simulink model "fractional_4"  (Simulink 7.4)
settings: Solver=ode45  StartTime=0.0  StopTime=1.6e-5  FixedStep=.01/(fr*N/M)  MaxStep=1/(25*fr*N)  RelTol=1e-5  AbsTol=1e-4
PreLoadFcn:
  | fr=10e6,fi=90e6,sen=10e6,N=10,M=.1
  | D=8;
StartFcn:
  | tic;
StopFcn:
  | trun=toc
undefined symbols (not defined in the file or in its folder): M, N, One, sen, sided
libraries: dspsigops x5, simulink_extras x5, dspsigattribs x4, simulink x3, dspstat3 x2, commblksprivate x2, dspsnks4 x1, dsparch4 x1
settings Model: Creator=rab  LastModifiedBy=Dick  BufferReuse=off
settings Model: ModifiedHistory=|
  | phase error compensation and swallow counter
  | incorporated by Benson,  Fall 2001.
settings DataIOCC: LimitDataPoints=off  SaveOutput=off  SaveTime=off  SignalLoggingName=sigsOut
settings OptimizationCC: BlockReduction=off  BooleanDataType=off  InlineInvariantSignals=on  OptimizeBlockIOStorage=off  BufferReuse=off  ExpressionFolding=off  LocalBlockOutputs=off  InitFltsAndDblsToZero=on
settings DebuggingCC: SaveWithParameterizedLinksMsg=none  SignalResolutionControl=TryResolveAllWithWarning  SolverPrmCheckMsg=none  MultiTaskDSMMsg=warning  MultiTaskCondExecSysMsg=none  StrictBusMsg=None
settings HardwareCC: TargetUnknown=on
settings RTWCC: IncludeERTFirstTime=on
settings GRTTargetCC: TargetFcnLib=ansi_tfl_tmw.mat

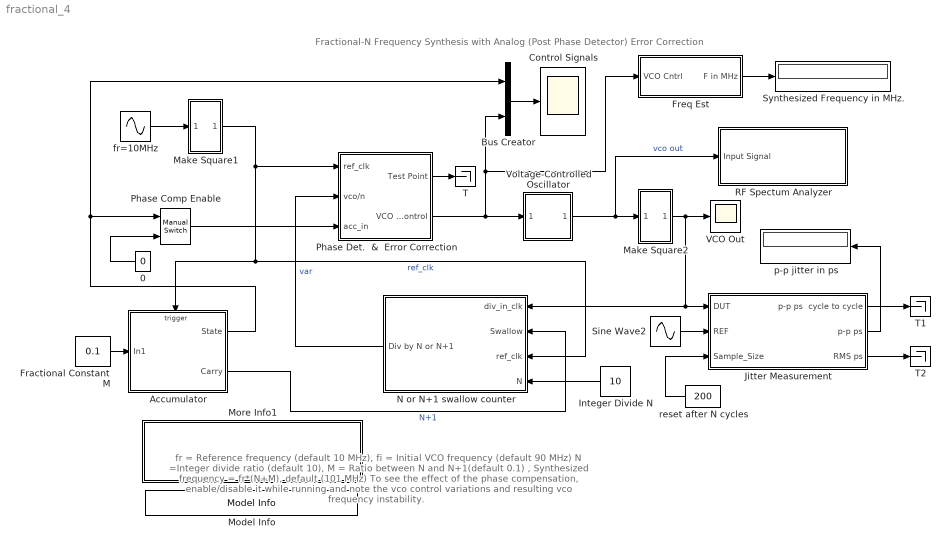
== system fractional_4 ==
  note: Fractional-N Frequency Synthesis with Analog (Post Phase Detector) Error Correction
  note: fr = Reference frequency (default 10 MHz),  fi = Initial VCO frequency (default 90 MHz)
      | N =Integer divide ratio (default 10),  M = Ratio between N and N+1(default 0.1) ,
      | Synthesized frequency = fr*(N+M), default (101 MHz)
      | To see the effect of the phase compensation, enable/disable it while running and note the vco control
      | variations and resulting vco frequency instability.
  0 : Constant  Value=0  OutDataType=sfix(16)  OutScaling=2^0
  Accumulator : Subsystem  TreatAsAtomicUnit=on
  Bus Creator : BusCreator  Inputs=2
  Control Signals : Scope
      settings: TimeRange=1.6e-005  YMin=-0.2  YMax=1.4  MaxDataPoints=60000
  Fractional Constant  M : Constant  Value=0.1  OutDataType=sfix(16)  OutScaling=2^0
  Freq Est : Subsystem
  Integer Divide N : Constant  Value=10  OutDataType=sfix(16)  OutScaling=2^0
  "Jitter Measurement " : Subsystem
  Make Square1 : Subsystem
      mask Type: Make Square
      mask Description:
      | For input +ve values output is 1
      | For input -ve values output is 0
      mask Display: plot(0,0,100,100,[90,70,70,50,50,30,30,10,10],[20,20,40,40,20,20,40,40,20],[90,87,84,80,76,73,70,67,63,60,57,53,50,47,44,40,36,33,30,27,23,20,17,13,10],[70,65,63,62,63,65,70,75,77,78,77,75,70,65,63,62,63,65,70,75,77,78,77,75,70])
  Make Square2 : Subsystem
      mask Type: Make Square
      mask Description:
      | For input +ve values output is 1
      | For input -ve values output is 0
      mask Display: plot(0,0,100,100,[90,70,70,50,50,30,30,10,10],[20,20,40,40,20,20,40,40,20],[90,87,84,80,76,73,70,67,63,60,57,53,50,47,44,40,36,33,30,27,23,20,17,13,10],[70,65,63,62,63,65,70,75,77,78,77,75,70,65,63,62,63,65,70,75,77,78,77,75,70])
  Model Info : simulink/Model-Wide Utilities/Model Info  SystemSampleTime=-1  InitialBlockCM=none  BlockCM=none  Frame=on  DisplayStringWithTags=Copywrite 2005-2010 The MathWorks, Inc.  HorizontalTextAlignment=Center  LeftAlignmentValue=0.5  SourceBlockDiagram=fractional_4  TagMaxNumber=20
  More Info1 : Subsystem
      mask Display: disp('Fractional N PLL with\n Analog Phase Correction\n Info ')
  N or N+1 swallow counter : Subsystem
  Phase Comp Enable : simulink/Signal Routing/Manual Switch  SystemSampleTime=-1  sw=1  action=0  varsize=off
  Phase Det.  &  Error Correction : Subsystem  mask{K=1.0}
      mask prompts: K "K="
      mask Display: disp('Phase Det')
  RF Spectum Analyzer : Subsystem  Description=Spectrum Analyzer  mask{BW=20e6, Fc=fr*(M+N)}
      mask prompts: BW "Bandwidth"; Fc "Center Freq"
      mask Display: fprintf('Spectrum Analyzer \n Fc=%7.2f MHz \n BW=%7.2f MHz',Fc/1e6,BW/1e6)
  Sine Wave2 : Sin  Amplitude=1  Bias=0  Frequency=2*pi*fr*(N+M)  Phase=0  Samples=10  SampleTime=0  Offset=0
  Synthesized Frequency in MHz. : Display
      settings: Decimation=401
  T : Terminator
  T1 : Terminator
  T2 : Terminator
  VCO Out : Scope
      settings: TimeRange=9.900990099009902e-009  YMin=-0.1  YMax=1.1  MaxDataPoints=500
  Voltage-Controlled Oscillator : Subsystem  mask(Voltage-Controlled Oscillator){Ac=1, Fc=fi, Kc=sen, Ph=0}
      mask prompts: Ac "Output amplitude:"; Fc "Oscillation frequency (Hz):"; Kc "Input sensitivity:"; Ph "Initial phase (rad):"
      mask help: Generate a continuous-time output signal whose frequency changes in response to the amplitude variations of the input signal. The input signal must be a sample-based scalar.
      mask init:
      | if ((length(Ac)~=1) | (length(Fc)~=1) | (length(Ph)~=1) | (length(Kc)~=1) )error('Mask parameters must be scalar values.');end;
      | pi2=2*pi;
      mask Help: helpview(commbhelp)
      mask Display: disp('VCO')
  fr=10MHz : Sin  Amplitude=1  Bias=0  Frequency=2*pi*fr  Phase=pi  Samples=10  SampleTime=0  Offset=0
  p-p jitter in ps : Display
  reset after N cycles : Constant  Value=200  VectorParams1D=off  OutDataType=sfix(16)  OutScaling=2^0
  wires:
  N or N+1 swallow counter/1(Div by N or N+1) -> Phase Det.  &  Error Correction/2(vco/n)  "var"
  Fractional Constant  M/1 -> Accumulator/1(In1)
  Make Square2/1(Out1) -> VCO Out/1, N or N+1 swallow counter/1(div_in_clk), "Jitter Measurement "/1(DUT)
  Accumulator/2(Carry) -> N or N+1 swallow counter/2(Swallow)  "N+1"
  Integer Divide N/1 -> N or N+1 swallow counter/4(N)
  0/1 -> Phase Comp Enable/2
  Freq Est/1(F in MHz) -> Synthesized Frequency in MHz./1
  Sine Wave2/1 -> "Jitter Measurement "/2(REF)
  "Jitter Measurement "/2(p-p ps) -> p-p jitter in ps/1
  reset after N cycles/1 -> "Jitter Measurement "/3(Sample_Size)
  Bus Creator/1 -> Control Signals/1
  Accumulator/1(State) -> Phase Comp Enable/1, Bus Creator/1
  Make Square1/1(Out1) -> Accumulator/Trigger, N or N+1 swallow counter/3(ref_clk), Phase Det.  &  Error Correction/1(ref_clk)  "ref_clk"
  Phase Comp Enable/1 -> Phase Det.  &  Error Correction/3("acc_in ")
  Voltage-Controlled Oscillator/1(out_1) -> Make Square2/1(In1), RF Spectum Analyzer/1(Input Signal)  "vco out"
  Phase Det.  &  Error Correction/2(VCO Control) -> Freq Est/1(VCO Cntrl), Bus Creator/2, Voltage-Controlled Oscillator/1(in_1)
  fr=10MHz/1 -> Make Square1/1(In1)
  Phase Det.  &  Error Correction/1(Test Point) -> T/1
  "Jitter Measurement "/1(p-p ps  cycle to cycle) -> T1/1
  "Jitter Measurement "/3(RMS ps) -> T2/1

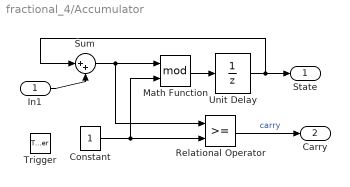
== system fractional_4/Accumulator ==
  In1 : Inport  OutDataType=sfix(16)  OutScaling=2^0
  Trigger : TriggerPort
  Constant : Constant  OutDataType=sfix(16)  OutScaling=2^0
  Math Function : Math  Operator=mod  OutDataType=sfix(16)  OutScaling=2^0  SaturateOnIntegerOverflow=on
  Relational Operator : RelationalOperator  InputSameDT=on
  Sum : Sum  Inputs=|++  OutDataType=sfix(16)  OutScaling=2^0  SaturateOnIntegerOverflow=on  InputSameDT=on  OutDataTypeStr=Inherit: Same as first input
  Unit Delay : UnitDelay  SampleTime=-1
  State : Outport  OutDataType=sfix(16)  OutScaling=2^0  InitialOutput=0
  Carry : Outport  Port=2  OutDataType=sfix(16)  OutScaling=2^0
  wires:
  In1/1 -> Sum/2
  Sum/1 -> Relational Operator/1, Math Function/1
  Math Function/1 -> Unit Delay/1
  Constant/1 -> Math Function/2, Relational Operator/2
  Relational Operator/1 -> Carry/1  "carry"
  Unit Delay/1 -> Sum/1, State/1

== system fractional_4/Freq Est ==
  VCO Cntrl : Inport  OutDataType=sfix(16)  OutScaling=2^0
  F : Constant  Value=fi  OutDataType=sfix(16)  OutScaling=2^0
  Gain1 : Gain  Gain=1e-6  ParameterDataType=sfix(16)  ParameterScaling=2^0  OutDataType=sfix(16)  OutScaling=2^0  SaturateOnIntegerOverflow=on  OutDataTypeStr=Inherit: Same as input  ParamDataTypeStr=Inherit: Same as input
  Gain3 : Gain  Gain=sen  ParameterDataType=sfix(16)  ParameterScaling=2^0  OutDataType=sfix(16)  OutScaling=2^0  SaturateOnIntegerOverflow=on  OutDataTypeStr=Inherit: Same as input  ParamDataTypeStr=Inherit: Same as input
  Sum1 : Sum  Inputs=|++  OutDataType=sfix(16)  OutScaling=2^0  SaturateOnIntegerOverflow=on  InputSameDT=on  OutDataTypeStr=Inherit: Same as first input
  F in MHz : Outport  OutDataType=sfix(16)  OutScaling=2^0
  wires:
  Sum1/1 -> Gain1/1
  F/1 -> Sum1/2
  Gain3/1 -> Sum1/1
  VCO Cntrl/1 -> Gain3/1
  Gain1/1 -> F in MHz/1

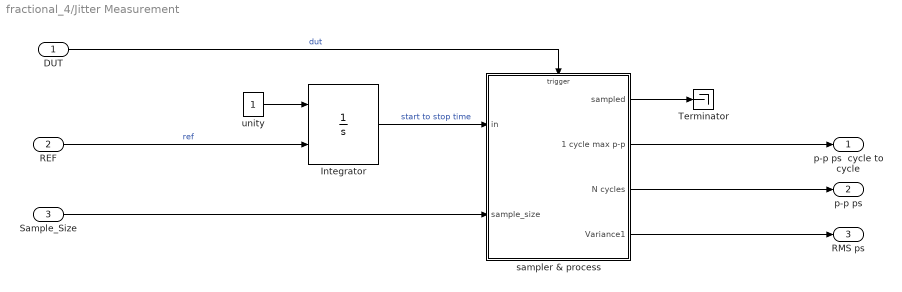
== system fractional_4/Jitter Measurement  ==
  DUT : Inport  OutDataType=sfix(16)  OutScaling=2^0
  REF : Inport  Port=2  OutDataType=sfix(16)  OutScaling=2^0
  Sample_Size : Inport  Port=3  OutDataType=sfix(16)  OutScaling=2^0
  Integrator : Integrator  ExternalReset=rising
  Terminator : Terminator
  sampler & process : Subsystem  TreatAsAtomicUnit=on
  unity : Constant  OutDataTypeMode=double  OutDataType=sfix(16)  OutScaling=2^0  OutDataTypeStr=double
  p-p ps  cycle to cycle : Outport  OutDataType=sfix(16)  OutScaling=2^0
  p-p ps : Outport  Port=2  OutDataType=sfix(16)  OutScaling=2^0
  RMS ps : Outport  Port=3  OutDataType=sfix(16)  OutScaling=2^0
  wires:
  DUT/1 -> sampler & process/Trigger  "dut"
  REF/1 -> Integrator/2  "ref"
  Integrator/1 -> sampler & process/1(in)  "start to stop time"
  Sample_Size/1 -> sampler & process/2(sample_size)
  sampler & process/3(N cycles) -> p-p ps/1
  sampler & process/4(Variance1) -> RMS ps/1
  unity/1 -> Integrator/1
  sampler & process/2(1 cycle max p-p) -> p-p ps  cycle to cycle/1
  sampler & process/1(sampled) -> Terminator/1

== system fractional_4/Make Square1 ==
  In1 : Inport  OutDataType=sfix(16)  OutScaling=2^0
  Constant : Constant  Value=0  OutDataType=sfix(16)  OutScaling=2^0
  Relational Operator : RelationalOperator  Operator=>  InputSameDT=on
  Out1 : Outport  OutDataType=sfix(16)  OutScaling=2^0
  wires:
  In1/1 -> Relational Operator/1
  Constant/1 -> Relational Operator/2
  Relational Operator/1 -> Out1/1

== system fractional_4/Make Square2 ==
  In1 : Inport  OutDataType=sfix(16)  OutScaling=2^0
  Constant : Constant  Value=0  OutDataType=sfix(16)  OutScaling=2^0
  Relational Operator : RelationalOperator  Operator=>  InputSameDT=on
  Out1 : Outport  OutDataType=sfix(16)  OutScaling=2^0
  wires:
  Relational Operator/1 -> Out1/1
  Constant/1 -> Relational Operator/2
  In1/1 -> Relational Operator/1

== system fractional_4/More Info1 ==
  note: Fractional-N PLL with Analog Phase Error Correction
  note: Fractional N PLL synthesizers attain improved frequency resolution at the expense
      | of increased circuit complexity and increased phase noise (timing jitter) over thier
      | non fractional counterparts. The average output frequency  of the PLL is (N+M)*fr where fr is
      | the frequency reference. The M term is the "fractional" part and lies between 0.0 and 1.
      |
      | This model implements a fractional N scheme with analog phase error correction
      | in the phase detector portion of the design. This *eliminates*  the sidebands introduced
      | by switching the loop divider between N and N+1.  Implementing the phase error correction
      | circuitry as part of the phase detector and loop compensation filter yeilds a design that
      | is easier to implement than the previous model that required a phase shifted clock.
      |
      |
      | 1)Phase-frequency detector and error compensator uses "dual D" flip flop phase
      | detector, integrator, sample / hold, and simple lead/lag loop filter.
      |
      | 2) Divide by N or N+1 is implemented using a "swallow" counter
      | scheme, like it would likely be done in hardware.
      |
      | 3) A modulo 1 accumulator controls the switching between N and N+1 with
      | the carry output.  The accumulator output (state) is used to drive the phase
      | compensation circuitry.
      |
      | 4) Run the simulation with the compensation off: switch in lower position.
      | Miminize the model to look at the graphs. Note the significant phase
      | jitter and sidebands due to the periodic variations of the VCO control
      | voltage.
      |
      | 5) Change the switch to the upper (compensation on) position. Note
      | the complete elimination  of  timing jitter, and, frequency spurs. Also note that
      | it is far easier to see the modulation in the frequency domain
      | sidebands  than the phase jitter of the clock.  The single remaining spur
      | (-100 dBc).
      |
      | 6) The Simulink model and simulation are virtually perfect. Real world component
      | limitations can now be introduced to study their effects on the system performance.

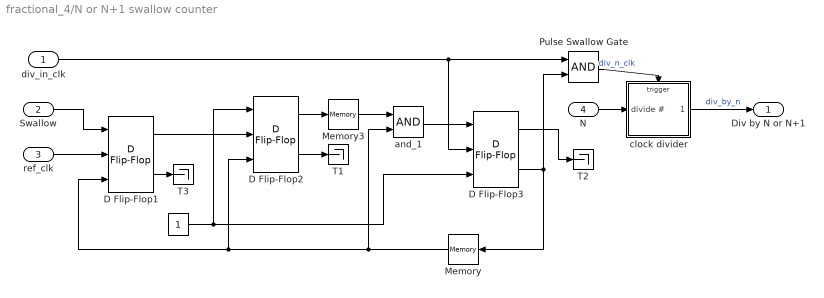
== system fractional_4/N or N+1 swallow counter ==
  div_in_clk : Inport  OutDataType=sfix(16)  OutScaling=2^0
  Swallow : Inport  Port=2  OutDataType=sfix(16)  OutScaling=2^0
  ref_clk : Inport  Port=3  OutDataType=sfix(16)  OutScaling=2^0
  N : Inport  Port=4  OutDataType=sfix(16)  OutScaling=2^0
  " " : Constant  OutDataType=sfix(16)  OutScaling=2^0
  D Flip-Flop1 : simulink_extras/Flip Flops/D Flip-Flop  SystemSampleTime=-1
  D Flip-Flop2 : simulink_extras/Flip Flops/D Flip-Flop  SystemSampleTime=-1
  D Flip-Flop3 : simulink_extras/Flip Flops/D Flip-Flop  SystemSampleTime=-1
  Memory : Memory
  Memory3 : Memory
  Pulse Swallow Gate : Logic
  T1 : Terminator
  T2 : Terminator
  T3 : Terminator
  and_1 : Logic
  clock divider : Subsystem  TreatAsAtomicUnit=on
  Div by N or N+1 : Outport  OutDataType=sfix(16)  OutScaling=2^0
  wires:
  N/1 -> clock divider/1("divide # ")
  D Flip-Flop1/2 -> T3/1
  D Flip-Flop2/2 -> T1/1
  D Flip-Flop3/1 -> T2/1
  Memory3/1 -> and_1/1
  D Flip-Flop1/1 -> D Flip-Flop2/2
  ref_clk/1 -> D Flip-Flop1/2
  Swallow/1 -> D Flip-Flop1/1
  and_1/1 -> D Flip-Flop3/1
  " "/1 -> D Flip-Flop3/3, D Flip-Flop2/1
  Memory/1 -> and_1/2, D Flip-Flop1/3, D Flip-Flop2/3
  D Flip-Flop3/2 -> Memory/1, Pulse Swallow Gate/2
  D Flip-Flop2/1 -> Memory3/1
  div_in_clk/1 -> D Flip-Flop3/2, Pulse Swallow Gate/1
  clock divider/1(" ") -> Div by N or N+1/1  "div_by_n"
  Pulse Swallow Gate/1 -> clock divider/Trigger  "div_n_clk"

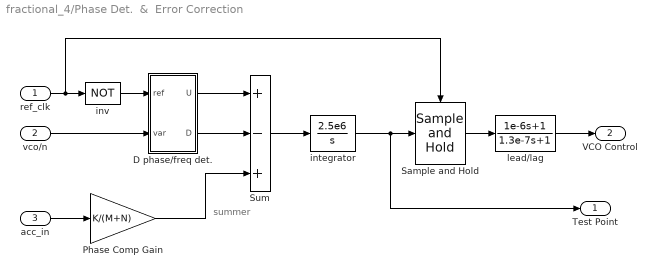
== system fractional_4/Phase Det.  &  Error Correction ==
  note: summer
  ref_clk : Inport  OutDataType=sfix(16)  OutScaling=2^0
  vco/n : Inport  Port=2  OutDataType=sfix(16)  OutScaling=2^0
  "acc_in " : Inport  Port=3  OutDataType=sfix(16)  OutScaling=2^0
  "D phase/freq det. " : Subsystem
  Phase Comp Gain : Gain  Gain=K/(M+N)  ParameterDataType=sfix(16)  ParameterScaling=2^0  OutDataType=sfix(16)  OutScaling=2^0  SaturateOnIntegerOverflow=on  OutDataTypeStr=Inherit: Same as input  ParamDataTypeStr=Inherit: Same as input
  Sample and Hold : dspsigops/Sample and Hold  SystemSampleTime=-1  trig=Rising edge  initCond=0  latchinput=off
  Sum : Sum  Inputs=+-+  OutDataType=sfix(16)  OutScaling=2^0  SaturateOnIntegerOverflow=on  InputSameDT=on  OutDataTypeStr=Inherit: Same as first input
  integrator : TransferFcn  Numerator=[2.5e6]  Denominator=[1 0]
  inv : Logic  Operator=NOT
  lead/lag : TransferFcn  Numerator=[1e-6 1]  Denominator=[1.3e-7 1]
  Test Point : Outport  OutDataType=sfix(16)  OutScaling=2^0
  VCO Control : Outport  Port=2  OutDataType=sfix(16)  OutScaling=2^0
  wires:
  "D phase/freq det. "/1(U) -> Sum/1
  "D phase/freq det. "/2(D) -> Sum/2
  Sum/1 -> integrator/1
  inv/1 -> "D phase/freq det. "/1(ref)
  ref_clk/1 -> inv/1, Sample and Hold/Trigger
  vco/n/1 -> "D phase/freq det. "/2(var)
  lead/lag/1 -> VCO Control/1
  "acc_in "/1 -> Phase Comp Gain/1
  Phase Comp Gain/1 -> Sum/3
  Sample and Hold/1 -> lead/lag/1
  integrator/1 -> Sample and Hold/1, Test Point/1

== system fractional_4/RF Spectum Analyzer ==
  Input Signal : Inport  OutDataType=sfix(16)  OutScaling=2^0
  Sine Wave1 : Sin  Amplitude=2*sqrt(2)  Bias=0  Frequency=2*pi*(Fc-BW/2)  Phase=-pi/2  Samples=10  SampleTime=0  Offset=0
  Spectrum Scope : dspsnks4/Spectrum Scope  DialogController=dspdialog.SpectrumScope  DialogControllerArgs=DataTag2  SystemSampleTime=-1  ScopeProperties=on  Domain=Frequency  HorizSpan=1  UseBuffer=on  BufferSize=256  Overlap=0  inpFftLenInherit=off  FFTlength=128  numAvg=1  DisplayProperties=off  AxisGrid=on  Memory=off  FrameNumber=on  AxisLegend=off  AxisZoom=off  OpenScopeAtSimStart=on  OpenScopeImmediately=off  FigPos=[12 34 389 175]  AxisProperties=off  XUnits=Hertz  XRange=One-sided ([0...Fs/2])  XDisplay=0  InheritXIncr=on  XIncr=1.0  XLabel=Samples  XLimit=Auto  YUnits=dBW  XMax=1  XMin=0  YLabel=dBW  LineProperties=off  wintypeSpecScope=Hann  RsSpecScope=50  betaSpecScope=5  winsampSpecScope=Periodic  XAxisParamsVer=6.9
      settings: YMin=-110  YMax=10
  anti alias : dsparch4/Analog Filter Design  method=Elliptic  filttype=Lowpass  N=8  Wlo=BW*2*pi  Whi=80  Rp=0.11  Rs=100
  down convert : Product  OutDataType=sfix(16)  OutScaling=2^0  SaturateOnIntegerOverflow=on  InputSameDT=on  OutDataTypeStr=Inherit: Same as first input
  sampler : ZeroOrderHold  SampleTime=1/(2.56*BW)
  wires:
  Sine Wave1/1 -> down convert/1
  sampler/1 -> Spectrum Scope/1
  anti alias/1 -> sampler/1
  down convert/1 -> anti alias/1
  Input Signal/1 -> down convert/2

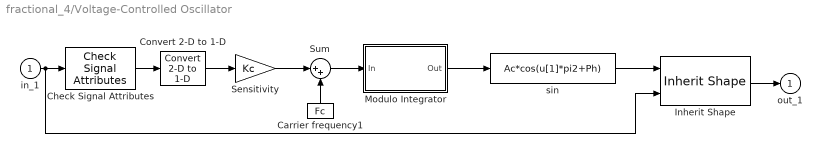
== system fractional_4/Voltage-Controlled Oscillator ==
  in_1 : Inport  OutDataType=sfix(16)  OutScaling=2^0
  Carrier frequency1 : Constant  Value=Fc  OutDataType=sfix(16)  OutScaling=2^0
  Check Signal Attributes : dspsigattribs/Check Signal Attributes  SystemSampleTime=-1  SigAttribCheckMethod=Does not match attributes exactly  Complexity=Ignore  Frame=Sample-based  DimsCheckMethod=Is...  Dimensions=Scalar (1-D or 2-D)  DatatypeCheckMethod=Ignore  DatatypeGeneral=Boolean  DtypeFloatSpecific=Any floating-point  DtypeFixedSpecific=Any fixed-point  DtypeIntSpecific=Any integer  SampleMode=Ignore
  Convert 2-D to 1-D : dspsigattribs/Convert 2-D to 1-D  SystemSampleTime=-1
  Inherit Shape : commblksprivate/Inherit Shape
  Modulo Integrator : Subsystem  mask(Modulo Integrator){modu=1, init=0}
      mask prompts: modu "Absolute value bound:"; init "Initial condition:"
      mask help:
      | Integrate the input signal in continuous time and then uses the Absolute value bound parameter, K, to produce output strictly between -K and K. The block uses the rem function in MATLAB.
      |
      | The input must be sample-based.
      mask init:
      | [modu, init]=commblkmodint(gcb);
      mask Help: helpview(commbhelp)
      mask Display: disp('Modulo\nIntegrator')
  Sensitivity : Gain  Gain=Kc  ParameterDataType=sfix(16)  ParameterScaling=2^0  OutDataType=sfix(16)  OutScaling=2^0  SaturateOnIntegerOverflow=on  OutDataTypeStr=Inherit: Same as input  ParamDataTypeStr=Inherit: Same as input
  Sum : Sum  Inputs=|++  OutDataType=sfix(16)  OutScaling=2^0  SaturateOnIntegerOverflow=on  InputSameDT=on  OutDataTypeStr=Inherit: Same as first input
  sin : Fcn  Expr=Ac*cos(u[1]*pi2+Ph)
  out_1 : Outport  OutDataType=sfix(16)  OutScaling=2^0
  wires:
  Sum/1 -> Modulo Integrator/1(In)
  Modulo Integrator/1(Out) -> sin/1
  Carrier frequency1/1 -> Sum/2
  Sensitivity/1 -> Sum/1
  in_1/1 -> Inherit Shape/2, Check Signal Attributes/1
  Convert 2-D to 1-D/1 -> Sensitivity/1
  sin/1 -> Inherit Shape/1
  Inherit Shape/1 -> out_1/1
  Check Signal Attributes/1 -> Convert 2-D to 1-D/1

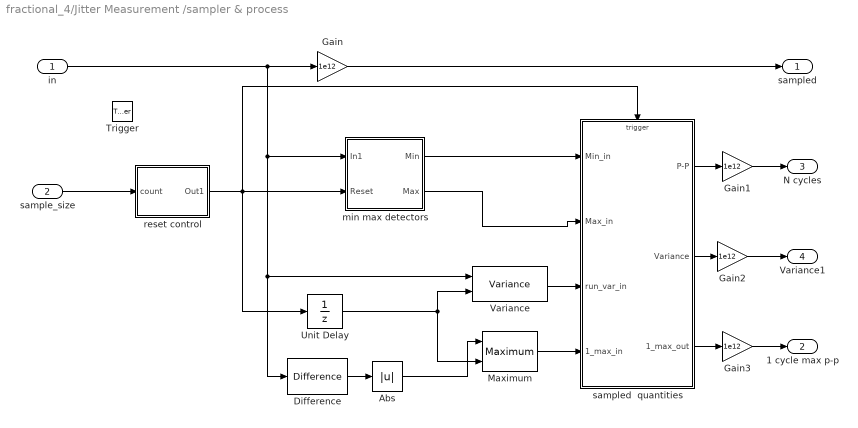
== system fractional_4/Jitter Measurement /sampler & process ==
  in : Inport  OutDataType=sfix(16)  OutScaling=2^0
  sample_size : Inport  Port=2  OutDataType=sfix(16)  OutScaling=2^0
  Trigger : TriggerPort
  Abs : Abs
  Difference : simulink/Discrete/Difference  SystemSampleTime=-1  ICPrevInput=0.0  OutMin=[]  OutMax=[]  OutDataType=sfix(16)  OutScaling=2^-10  DoSatur=off
  Gain{,1..3} (4 alike) : Gain  Gain=1e12  ParameterDataType=sfix(16)  ParameterScaling=2^0  OutDataType=sfix(16)  OutScaling=2^0
  Maximum : dspstat3/Maximum  DialogController=dspDDGCreate  DialogControllerArgs=DataTag0  fcn=Running  reset=Rising edge  indexBase=One  operateOver=Each column  Dimension=1  colComp=on  operation=maximum  roiEnable=off  roiType=Rectangles  roiPortion=Entire ROI  roiOutput=Individual statistics for each ROI  roiFlag=off  accumDataTypeStr=Inherit: Same as product output  accumLastDataTypeStr=Inherit: Same as product output  roundingMode=Floor  overflowMode=off
  Unit Delay : UnitDelay  SampleTime=-1
  Variance : dspstat3/Variance  DialogController=dspDDGCreate  DialogControllerArgs=DataTag1  run=on  reset_popup=Rising edge  directionMode=Each column  dimension=1  treatSBRowAsCol=on  roiEnable=off  roiType=Rectangles  roiPortion=Entire ROI  roiOutput=Individual statistics for each ROI  roiFlag=off  roundingMode=Floor  overflowMode=off
  min max detectors : Subsystem
  reset control : Subsystem
  sampled  quantities : Subsystem  TreatAsAtomicUnit=on
  sampled : Outport  OutDataType=sfix(16)  OutScaling=2^0
  1 cycle max p-p : Outport  Port=2  OutDataType=sfix(16)  OutScaling=2^0
  N cycles : Outport  Port=3  OutDataType=sfix(16)  OutScaling=2^0
  Variance1 : Outport  Port=4  OutDataType=sfix(16)  OutScaling=2^0
  wires:
  in/1 -> Gain/1, Variance/1, Difference/1, min max detectors/1(In1)
  Difference/1 -> Abs/1
  Abs/1 -> Maximum/1
  sample_size/1 -> reset control/1(count)
  reset control/1(Out1) -> Unit Delay/1, sampled  quantities/Trigger, min max detectors/2(Reset)
  sampled  quantities/1(P-P) -> Gain1/1
  Variance/1 -> sampled  quantities/3(run_var_in)
  sampled  quantities/2(Variance) -> Gain2/1
  Unit Delay/1 -> Variance/2, Maximum/2
  Maximum/1 -> sampled  quantities/4(1_max_in)
  sampled  quantities/3(1_max_out) -> Gain3/1
  Gain/1 -> sampled/1
  Gain1/1 -> N cycles/1
  Gain2/1 -> Variance1/1
  Gain3/1 -> 1 cycle max p-p/1
  min max detectors/2(Max) -> sampled  quantities/2(Max_in)
  min max detectors/1(Min) -> sampled  quantities/1(Min_in)

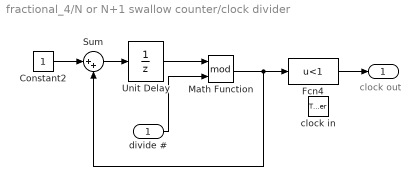
== system fractional_4/N or N+1 swallow counter/clock divider ==
  note: clock out
  "divide # " : Inport  OutDataType=sfix(16)  OutScaling=2^0
  clock in : TriggerPort
  Constant2 : Constant  OutDataType=sfix(16)  OutScaling=2^0
  Fcn4 : Fcn  Expr=u<1
  Math Function : Math  Operator=mod  OutDataType=sfix(16)  OutScaling=2^0  SaturateOnIntegerOverflow=on
  Sum : Sum  Inputs=|++  OutDataType=sfix(16)  OutScaling=2^0  SaturateOnIntegerOverflow=on  InputSameDT=on  OutDataTypeStr=Inherit: Same as first input
  Unit Delay : UnitDelay  SampleTime=-1
  " " : Outport  OutDataType=sfix(16)  OutScaling=2^0
  wires:
  "divide # "/1 -> Math Function/2
  Fcn4/1 -> " "/1
  Math Function/1 -> Fcn4/1, Sum/2
  Unit Delay/1 -> Math Function/1
  Constant2/1 -> Sum/1
  Sum/1 -> Unit Delay/1

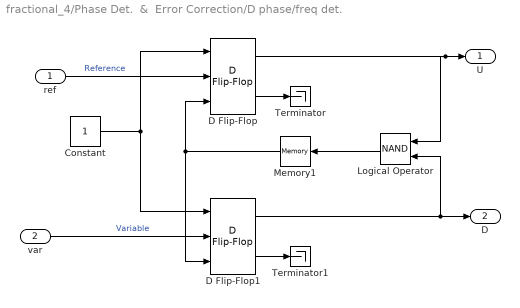
== system fractional_4/Phase Det.  &  Error Correction/D phase/freq det.  ==
  ref : Inport  OutDataType=sfix(16)  OutScaling=2^0
  var : Inport  Port=2  OutDataType=sfix(16)  OutScaling=2^0
  Constant : Constant  OutDataType=sfix(16)  OutScaling=2^0
  D Flip-Flop : simulink_extras/Flip Flops/D Flip-Flop  SystemSampleTime=-1
  D Flip-Flop1 : simulink_extras/Flip Flops/D Flip-Flop  SystemSampleTime=-1
  Logical Operator : Logic  Operator=NAND
  Memory1 : Memory
  Terminator : Terminator
  Terminator1 : Terminator
  U : Outport  OutDataType=sfix(16)  OutScaling=2^0
  D : Outport  Port=2  OutDataType=sfix(16)  OutScaling=2^0
  wires:
  var/1 -> D Flip-Flop1/2  "Variable"
  D Flip-Flop/2 -> Terminator/1
  D Flip-Flop1/2 -> Terminator1/1
  ref/1 -> D Flip-Flop/2  "Reference"
  Constant/1 -> D Flip-Flop/1, D Flip-Flop1/1
  Memory1/1 -> D Flip-Flop/3, D Flip-Flop1/3
  D Flip-Flop/1 -> U/1, Logical Operator/1
  D Flip-Flop1/1 -> D/1, Logical Operator/2
  Logical Operator/1 -> Memory1/1

== system fractional_4/Voltage-Controlled Oscillator/Modulo Integrator ==
  In : Inport  OutDataType=sfix(16)  OutScaling=2^0
  "Exclude Frame-based Input " : dspsigattribs/Check Signal Attributes  SystemSampleTime=-1  SigAttribCheckMethod=Matches attributes exactly  Complexity=Ignore  Frame=Frame-based  DimsCheckMethod=Ignore  Dimensions=Scalar (1-D or 2-D)  DatatypeCheckMethod=Ignore  DatatypeGeneral=Boolean  DtypeFloatSpecific=Any floating-point  DtypeFixedSpecific=Any fixed-point  DtypeIntSpecific=Any integer  SampleMode=Ignore
  Exclude Full Matrix : dspsigattribs/Check Signal Attributes  SystemSampleTime=-1  SigAttribCheckMethod=Matches attributes exactly  Complexity=Ignore  Frame=Ignore  DimsCheckMethod=Is...  Dimensions=Full matrix (2-D)  DatatypeCheckMethod=Ignore  DatatypeGeneral=Boolean  DtypeFloatSpecific=Any floating-point  DtypeFixedSpecific=Any fixed-point  DtypeIntSpecific=Any integer  SampleMode=Ignore
  Inherit Shape : commblksprivate/Inherit Shape
  Modulo Integrator : Subsystem
  Out : Outport  OutDataType=sfix(16)  OutScaling=2^0
  wires:
  Exclude Full Matrix/1 -> "Exclude Frame-based Input "/1
  "Exclude Frame-based Input "/1 -> Modulo Integrator/1(In1)
  In/1 -> Exclude Full Matrix/1, Inherit Shape/2
  Modulo Integrator/1(Out1) -> Inherit Shape/1
  Inherit Shape/1 -> Out/1

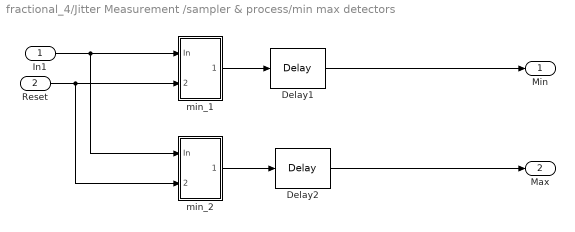
== system fractional_4/Jitter Measurement /sampler & process/min max detectors ==
  In1 : Inport  OutDataType=sfix(16)  OutScaling=2^0
  Reset : Inport  Port=2  OutDataType=sfix(16)  OutScaling=2^0
  Delay1 : dspsigops/Delay  dly_unit=Samples  delay=1  ic_detail=off  dif_ic_for_ch=off  dif_ic_for_dly=off  ic=0  reset_popup=None
  Delay2 : dspsigops/Delay  dly_unit=Samples  delay=1  ic_detail=off  dif_ic_for_ch=off  dif_ic_for_dly=off  ic=0  reset_popup=None
  min_1 : Subsystem
  min_2 : Subsystem
  Min : Outport  OutDataType=sfix(16)  OutScaling=2^0
  Max : Outport  Port=2  OutDataType=sfix(16)  OutScaling=2^0
  wires:
  Reset/1 -> min_1/2(Rst), min_2/2(Rst)
  In1/1 -> min_1/1(In), min_2/1(In)
  min_1/1(Out) -> Delay1/1
  min_2/1(Out) -> Delay2/1
  Delay1/1 -> Min/1
  Delay2/1 -> Max/1

== system fractional_4/Jitter Measurement /sampler & process/reset control ==
  count : Inport  OutDataType=sfix(16)  OutScaling=2^0
  Constant2 : Constant  OutDataType=sfix(16)  OutScaling=2^0
  Fcn4 : Fcn  Expr=u<1
  Math Function : Math  Operator=mod  OutDataType=sfix(16)  OutScaling=2^0  SaturateOnIntegerOverflow=on
  Sum2 : Sum  Inputs=|++  OutDataType=sfix(16)  OutScaling=2^0  SaturateOnIntegerOverflow=on  InputSameDT=on  OutDataTypeStr=Inherit: Same as first input
  Unit Delay1 : UnitDelay  SampleTime=-1
  Out1 : Outport  OutDataType=sfix(16)  OutScaling=2^0
  wires:
  Math Function/1 -> Fcn4/1, Sum2/2
  Unit Delay1/1 -> Math Function/1
  Constant2/1 -> Sum2/1
  Sum2/1 -> Unit Delay1/1
  Fcn4/1 -> Out1/1
  count/1 -> Math Function/2

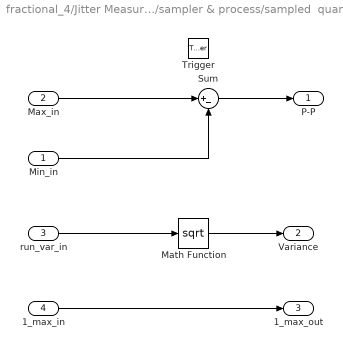
== system fractional_4/Jitter Measurement /sampler & process/sampled  quantities ==
  Min_in : Inport  OutDataType=sfix(16)  OutScaling=2^0
  Max_in : Inport  Port=2  OutDataType=sfix(16)  OutScaling=2^0
  run_var_in : Inport  Port=3  OutDataType=sfix(16)  OutScaling=2^0
  1_max_in : Inport  Port=4  OutDataType=sfix(16)  OutScaling=2^0
  Trigger : TriggerPort
  Math Function : Math  Operator=sqrt  OutDataType=sfix(16)  OutScaling=2^0  SaturateOnIntegerOverflow=on
  Sum : Sum  Inputs=|+-  OutDataType=sfix(16)  OutScaling=2^0  SaturateOnIntegerOverflow=on  InputSameDT=on  OutDataTypeStr=Inherit: Same as first input
  P-P : Outport  OutDataType=sfix(16)  OutScaling=2^0
  Variance : Outport  Port=2  OutDataType=sfix(16)  OutScaling=2^0
  1_max_out : Outport  Port=3  OutDataType=sfix(16)  OutScaling=2^0
  wires:
  Max_in/1 -> Sum/1
  Min_in/1 -> Sum/2
  Sum/1 -> P-P/1
  Math Function/1 -> Variance/1
  run_var_in/1 -> Math Function/1
  1_max_in/1 -> 1_max_out/1

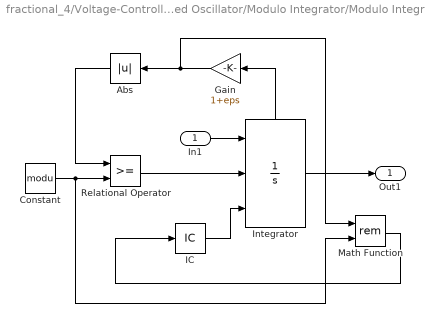
== system fractional_4/Voltage-Controlled Oscillator/Modulo Integrator/Modulo Integrator ==
  In1 : Inport  OutDataType=sfix(16)  OutScaling=2^0
  Abs : Abs  OutDataType=sfix(16)  OutScaling=2^0  SaturateOnIntegerOverflow=on
  Constant : Constant  Value=modu  OutDataType=sfix(16)  OutScaling=2^0
  Gain : Gain  Gain=1+eps  ParameterDataType=sfix(16)  ParameterScaling=2^0  OutDataType=sfix(16)  OutScaling=2^0  SaturateOnIntegerOverflow=on  OutDataTypeStr=Inherit: Same as input  ParamDataTypeStr=Inherit: Same as input
  IC : InitialCondition  Value=init
  Integrator : Integrator  ExternalReset=rising  InitialConditionSource=external  UpperSaturationLimit=1  LowerSaturationLimit=0  ShowStatePort=on
  Math Function : Math  Operator=rem  OutDataType=sfix(16)  OutScaling=2^0  SaturateOnIntegerOverflow=on
  Relational Operator : RelationalOperator  InputSameDT=on
  Out1 : Outport  OutDataType=sfix(16)  OutScaling=2^0
  wires:
  IC/1 -> Integrator/3
  In1/1 -> Integrator/1
  Integrator/1 -> Out1/1
  Math Function/1 -> IC/1
  Abs/1 -> Relational Operator/1
  Relational Operator/1 -> Integrator/2
  Constant/1 -> Math Function/2, Relational Operator/2
  Integrator/State -> Gain/1
  Gain/1 -> Abs/1, Math Function/1

== system fractional_4/Jitter Measurement /sampler & process/min max detectors/min_1 ==
  In : Inport  OutDataType=sfix(16)  OutScaling=2^0
  Rst : Inport  Port=2  OutDataType=sfix(16)  OutScaling=2^0
  Delay : dspsigops/Delay  dly_unit=Samples  delay=1  ic_detail=off  dif_ic_for_ch=off  dif_ic_for_dly=off  ic=1e6  reset_popup=Non-zero sample
  Relational Operator : RelationalOperator  Operator=<  LogicOutDataTypeMode=boolean  OutDataTypeStr=boolean
  Switch : Switch  Threshold=.5
  Out : Outport  OutDataType=sfix(16)  OutScaling=2^0
  wires:
  In/1 -> Relational Operator/1, Switch/1
  Rst/1 -> Delay/2
  Delay/1 -> Relational Operator/2, Switch/3
  Relational Operator/1 -> Switch/2
  Switch/1 -> Delay/1, Out/1

== system fractional_4/Jitter Measurement /sampler & process/min max detectors/min_2 ==
  In : Inport  OutDataType=sfix(16)  OutScaling=2^0
  Rst : Inport  Port=2  OutDataType=sfix(16)  OutScaling=2^0
  Delay : dspsigops/Delay  dly_unit=Samples  delay=1  ic_detail=off  dif_ic_for_ch=off  dif_ic_for_dly=off  ic=-1e6  reset_popup=Non-zero sample
  Relational Operator : RelationalOperator  Operator=>  LogicOutDataTypeMode=boolean  OutDataTypeStr=boolean
  Switch : Switch  Threshold=.5
  Out : Outport  OutDataType=sfix(16)  OutScaling=2^0
  wires:
  Switch/1 -> Out/1, Delay/1
  Relational Operator/1 -> Switch/2
  Delay/1 -> Switch/3, Relational Operator/2
  Rst/1 -> Delay/2
  In/1 -> Switch/1, Relational Operator/1
